simulink model "EScooterBMS"  (R2025b)
settings: Solver=VariableStepAuto  StartTime=0.0  StopTime=3600*20  RelTol=1e-3
InitFcn:
  | EScooterBMS_params
undefined symbols (not defined in the file): balancingThreshold, battery_builder_rtmsupport, CC_Current, currentThreshold, CV_gain, dischargeCurrent, gcbh, initialSOC, initialSOCGuess, noisePower, R, Ts, voltageMin, voltageThreshold
libraries: nesl_utility x6, simulink x5, fl_lib x5, MA1865_1RC_Balancing_lib x2, BatteryBalancing x1, BatteryEstimators x1
settings Model: PacingRate=100  Creator=sturton  LastModifiedBy=sturton

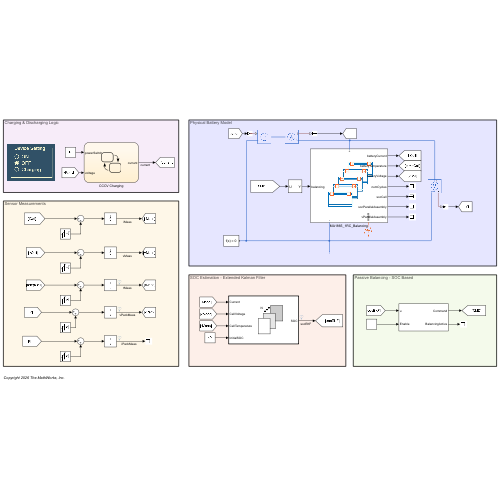
[thumbnail: Simulink's stored preview of the top-level diagram]
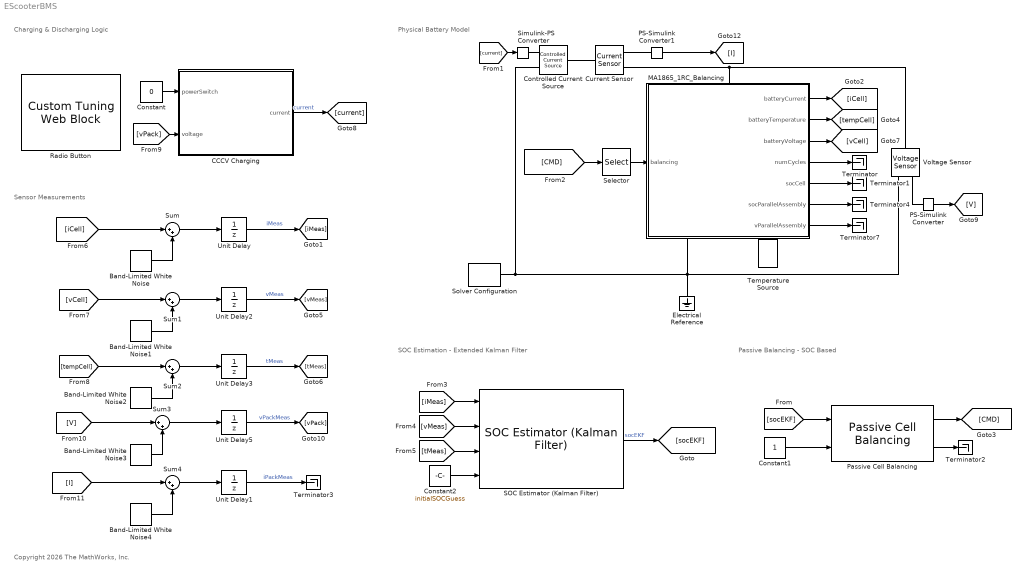
== system EScooterBMS ==
  note: Copyright 2026 The MathWorks, Inc.
  note: Charging & Discharging Logic
  note: Sensor Measurements
  note: SOC Estimation - Extended Kalman Filter
  note: Physical Battery Model
  note: Passive Balancing - SOC Based
  Band-Limited White Noise : simulink/Sources/Band-Limited White Noise  Cov=noisePower  Ts=Ts  seed=[23341]
  Band-Limited White Noise1 : simulink/Sources/Band-Limited White Noise  Cov=noisePower/100;  Ts=Ts  seed=[23341]
  Band-Limited White Noise2 : simulink/Sources/Band-Limited White Noise  Cov=noisePower  Ts=Ts  seed=[23341]
  Band-Limited White Noise3 : simulink/Sources/Band-Limited White Noise  Cov=noisePower/100;  Ts=Ts  seed=[23341]
  Band-Limited White Noise4 : simulink/Sources/Band-Limited White Noise  Cov=noisePower  Ts=Ts  seed=[23341]
  CCCV Charging : Stateflow chart  TreatAsAtomicUnit=on
  Constant : Constant  Value=0
  Constant1 : Constant
  Constant2 : Constant  Value=initialSOCGuess
  Controlled Current Source : fl_lib/Electrical/Electrical Sources/Controlled Current Source
  Current Sensor : fl_lib/Electrical/Electrical Sensors/Current Sensor
  Electrical Reference : fl_lib/Electrical/Electrical Elements/Electrical Reference
  MA1865_1RC_Balancing : Subsystem  LoadFcn=battery_builder_rtmsupport('loadfcn',gcbh);
      settings: CopyFcn=battery_builder_rtmsupport('copyfcn',gcbh);  PreCopyFcn=battery_builder_rtmsupport('precopyfcn',gcbh);  PreDeleteFcn=battery_builder_rtmsupport('predeletefcn',gcbh);  PortSchema="{\"entries\":[{\"content\":{\"sides\":[{\"content\":{\"connectorIds\":[\"LConn1\"]},\"type\":\"ConnectorPlacement.EquallySpacedRectSide\",\"uuid\":\"68ab6467-2481-45d5-b31e-65f7da693cdd\"},{\"content\":{\"connectorIds\":[\"RConn1\",\"RConn2\"],\"side\":\"RIGHT\"},\"type\":\"ConnectorPlacement.EquallySpacedRectSide\",\"uuid\":\"28f8b7ad-849b-43ef-a357-ff2296ceb517\"},{\"content\":{\"connectorIds\":[\"In1\"],\"side\":\"TOP\"},\"type\":\"ConnectorPlacement.EquallySpacedRectSide\",\"uuid\":\"4bc70995-0dac-442d-9c06-590b4a7fbec4\"},{\"content\":{\"connectorIds\":[\"Out1\",\"Out2\",\"Out3\",\"Out4\",\"Out5\",\"Out6\",\"Out7\"],\"side\":\"BOTTOM\"},\"type\":\"ConnectorPlacement.EquallySpacedRectSide\",\"uuid\":\"3fb7c4af-3c1e-4317-a54e-7f7a844b4b32\"}]},\"type\":\"ConnectorPlacement.EquallySpacedConnector\",\"uuid\":\"b72d0926-0e23-41a7-8fa8-9d2afaa8a9c6\"}],\"packageUris\":[\"http://schema.mathworks.com/mf0/Connector/R2020b\"],\"version\":\"1.0\"}"
      mask Display: image('$imagefile')
  PS-Simulink Converter : nesl_utility/PS-Simulink Converter  PhysicalDomain=network_engine_domain  SubClassName=ps_output  LeftPortType=input  RightPortType=output  PseudoPeriodic=off  Frequencies=[]  VectorFormat=inherit  Unit=inherit  AffineConversion=off
  PS-Simulink Converter1 : nesl_utility/PS-Simulink Converter  PhysicalDomain=network_engine_domain  SubClassName=ps_output  LeftPortType=input  RightPortType=output  PseudoPeriodic=off  Frequencies=[]  VectorFormat=inherit  Unit=inherit  AffineConversion=off
  Passive Cell Balancing : BatteryBalancing/Passive Cell Balancing  Threshold=balancingThreshold  HysteresisBand=0  Td_on=1  Td_off=1  Ts=Ts  dataType=double
      settings: LibrarySourceBlock=batt_sl_lib/Cell Balancing/Passive Cell Balancing
  Radio Button : CustomTuningWebBlock  LabelPosition=Hide  ShowInitialText=on  Configuration="{\"components\":[{\"name\":\"RadioButtonStateComponent\",\"settings\":{\"clearedIcon\":{\"size\":[1,1],\"src\":\"data:image\\/svg+xml;base64,PD94bWwgdmVyc2lvbj0iMS4wIiBlbmNvZGluZz0iVVRGLTgiPz4KPHN2ZyBpZD0ic3ZnOCIgeG1sbnM9Imh0dHA6Ly93d3cudzMub3JnLzIwMDAvc3ZnIiB2ZXJzaW9uPSIxLjEiIHhtbG5zOmNjPSJodHRwOi8vY3JlYXRpdmVjb21tb25zLm9yZy9ucyMiIHhtbG5zOmRjPSJodHRwOi8vcHVybC5vcmcvZGMvZWxlbWVudHMvMS4xLyIgeG1sbnM6aW5rc2NhcGU9Imh0dHA6Ly93d3cuaW5rc2NhcGUub3JnL25hbWVzcGFjZXMvaW5rc2NhcGUiIHhtbG5zOnJkZj0iaHR0cDovL3d3dy53My5vcmcvMTk5OS8wMi8yMi1yZGYtc3ludGF4LW5zIyIgeG1sbnM6c29kaXBvZGk9Imh0dHA6Ly9zb2RpcG9kaS5zb3VyY2Vmb3JnZS5uZXQvRFREL3NvZGlwb2RpLTAuZHRkIiB4bWxuczpzdmc9Imh0dHA6Ly93d3cudzMub3JnLzIwMDAvc3ZnIiB2aWV3Qm94PSIwIDAgMzE2LjQgMzE2LjQiPgogIDwhLS0gR2VuZXJhdG9yOiBBZG9iZSBJbGx1c3RyYXRvciAyOS4xLjAsIFNWRyBFeHBvcnQgUGx1Zy1JbiAuIFNWRyBWZXJzaW9uOiAyLjEuMCBCdWlsZCAxNDIpICAtLT4KICA8ZGVmcz4KICAgIDxzdHlsZT4KICAgICAgLnN0MCB7CiAgICAgICAgZmlsbDogbm9uZTsKICAgICAgICBzdHJva2Utd2lkdGg6IDMwcHg7CiAgICAgIH0KCiAgICAgIC5zdDAsIC5zdDEgewogICAgICAgIHN0cm9rZTogI2ZjZmNjNTsKICAgICAgICBzdHJva2UtbWl0ZXJsaW1pdDogMTEuMzsKICAgICAgfQoKICAgICAgLnN0MSB7CiAgICAgICAgZGlzcGxheTogbm9uZTsKICAgICAgICBmaWxsOiAjZmNmY2M1OwogICAgICB9CiAgICA8L3N0eWxlPgogIDwvZGVmcz4KICA8c29kaXBvZGk6bmFtZWR2aWV3IGlkPSJiYXNlIiBib3JkZXJjb2xvcj0iIzY2NjY2NiIgYm9yZGVyb3BhY2l0eT0iMS4wIiBpbmtzY2FwZTpjdXJyZW50LWxheWVyPSJsYXllcjEiIGlua3NjYXBlOmN4PSI0MDAiIGlua3NjYXBlOmN5PSI1NjAiIGlua3NjYXBlOmRvY3VtZW50LXJvdGF0aW9uPSIwIiBpbmtzY2FwZTpkb2N1bWVudC11bml0cz0ibW0iIGlua3NjYXBlOnBhZ2VvcGFjaXR5PSIwLjAiIGlua3NjYXBlOnBhZ2VzaGFkb3c9IjIiIGlua3NjYXBlOndpbmRvdy1oZWlnaHQ9IjEwODEiIGlua3NjYXBlOndpbmRvdy1tYXhpbWl6ZWQ9IjAiIGlua3NjYXBlOndpbmRvdy13aWR0aD0iMTI1MiIgaW5rc2NhcGU6d2luZG93LXg9IjAiIGlua3NjYXBlOndpbmRvdy15PSIyMyIgaW5rc2NhcGU6em9vbT0iMC4zNSIgcGFnZWNvbG9yPSIjZmZmZmZmIiBzaG93Z3JpZD0iZmFsc2UiLz4KICA8Y2lyY2xlIGNsYXNzPSJzdDAiIGN4PSIxNTguMiIgY3k9IjE1OC4yIiByPSIxMzYiLz4KICA8Y2lyY2xlIGNsYXNzPSJzdDEiIGN4PSIxNTguMiIgY3k9IjE1OC4yIiByPSI5OS42Ii8+Cjwvc3ZnPg==\"},\"color\":[0,0,0],\"groupBorderColor\":[252,252,197],\"groupBorderThickness\":\"1\",\"groupTitle\":\"Device Setting\",\"iconOffset\":\"0.5\",\"iconPlacement\":\"left\",\"labelOffset\":[0.2,0.1],\"position\":[0,0,1,1],\"selectedIcon\":{\"size\":[1,1],\"src\":\"data:image\\/svg+xml;base64,PD94bWwgdmVyc2lvbj0iMS4wIiBlbmNvZGluZz0iVVRGLTgiPz4KPHN2ZyBpZD0ic3ZnOCIgeG1sbnM9Imh0dHA6Ly93d3cudzMub3JnLzIwMDAvc3ZnIiB2ZXJzaW9uPSIxLjEiIHhtbG5zOmNjPSJodHRwOi8vY3JlYXRpdmVjb21tb25zLm9yZy9ucyMiIHhtbG5zOmRjPSJodHRwOi8vcHVybC5vcmcvZGMvZWxlbWVudHMvMS4xLyIgeG1sbnM6aW5rc2NhcGU9Imh0dHA6Ly93d3cuaW5rc2NhcGUub3JnL25hbWVzcGFjZXMvaW5rc2NhcGUiIHhtbG5zOnJkZj0iaHR0cDovL3d3dy53My5vcmcvMTk5OS8wMi8yMi1yZGYtc3ludGF4LW5zIyIgeG1sbnM6c29kaXBvZGk9Imh0dHA6Ly9zb2RpcG9kaS5zb3VyY2Vmb3JnZS5uZXQvRFREL3NvZGlwb2RpLTAuZHRkIiB4bWxuczpzdmc9Imh0dHA6Ly93d3cudzMub3JnLzIwMDAvc3ZnIiB2aWV3Qm94PSIwIDAgMzE2LjQgMzE2LjQiPgogIDwhLS0gR2VuZXJhdG9yOiBBZG9iZSBJbGx1c3RyYXRvciAyOS4xLjAsIFNWRyBFeHBvcnQgUGx1Zy1JbiAuIFNWRyBWZXJzaW9uOiAyLjEuMCBCdWlsZCAxNDIpICAtLT4KICA8ZGVmcz4KICAgIDxzdHlsZT4KICAgICAgLnN0MCB7CiAgICAgICAgZmlsbDogI2ZjZmNjNTsKICAgICAgfQoKICAgICAgLnN0MCwgLnN0MSB7CiAgICAgICAgc3Ryb2tlOiAjZmNmY2M1OwogICAgICAgIHN0cm9rZS1taXRlcmxpbWl0OiAxMS4zOwogICAgICB9CgogICAgICAuc3QxIHsKICAgICAgICBmaWxsOiBub25lOwogICAgICAgIHN0cm9rZS13aWR0aDogMzBweDsKICAgICAgfQogICAgPC9zdHlsZT4KICA8L2RlZnM+CiAgPHNvZGlwb2RpOm5hbWVkdmlldyBpZD0iYmFzZSIgYm9yZGVyY29sb3I9IiM2NjY2NjYiIGJvcmRlcm9wYWNpdHk9IjEuMCIgaW5rc2NhcGU6Y3VycmVudC1sYXllcj0ibGF5ZXIxIiBpbmtzY2FwZTpjeD0iNDAwIiBpbmtzY2FwZTpjeT0iNTYwIiBpbmtzY2FwZTpkb2N1bWVudC1yb3RhdGlvbj0iMCIgaW5rc2NhcGU6ZG9jdW1lbnQtdW5pdHM9Im1tIiBpbmtzY2FwZTpwYWdlb3BhY2l0eT0iMC4wIiBpbmtzY2FwZTpwYWdlc2hhZG93PSIyIiBpbmtzY2FwZTp3aW5kb3ctaGVpZ2h0PSIxMDgxIiBpbmtzY2FwZTp3aW5kb3ctbWF4aW1pemVkPSIwIiBpbmtzY2FwZTp3aW5kb3ctd2lkdGg9IjEyNTIiIGlua3NjYXBlOndpbmRvdy14PSIwIiBpbmtzY2FwZTp3aW5kb3cteT0iMjMiIGlua3NjYXBlOnpvb209IjAuMzUiIHBhZ2Vjb2xvcj0iI2ZmZmZmZiIgc2hvd2dyaWQ9ImZhbHNlIi8+CiAgPGNpcmNsZSBjbGFzcz0ic3QxIiBjeD0iMTU4LjIiIGN5PSIxNTguMiIgcj0iMTM2Ii8+CiAgPGNpcmNsZSBjbGFzcz0ic3QwIiBjeD0iMTU4LjIiIGN5PSIxNTguMiIgcj0iOTkuNiIvPgo8L3N2Zz4=\"},\"showGroup\":true,\"states\":[{\"Label\":{\"show\":true,\"text\":{\"content\":\"ON\",\"font\":\"Helvetica\"}},\"Value\":1},{\"Label\":{\"show\":true,\"text\":{\"content\":\"OFF\",\"font\":\"Helvetica\"}},\"Value\":0},{\"Label\":{\"show\":true,\"text\":{\"content\":\"Charging\",\"font\":\"Helvetica\"}},\"Value\":2}]}},{\"name\":\"BackgroundImageComponent\",\"settings\":{\"image\":{\"size\":[146,150],\"src\":\"data:image\\/svg+xml;base64,PD94bWwgdmVyc2lvbj0iMS4wIiBlbmNvZGluZz0iVVRGLTgiPz4KPHN2ZyBpZD0iZnJhbWUiIHhtbG5zPSJodHRwOi8vd3d3LnczLm9yZy8yMDAwL3N2ZyIgdmVyc2lvbj0iMS4xIiB4bWxuczp4bGluaz0iaHR0cDovL3d3dy53My5vcmcvMTk5OS94bGluayIgdmlld0JveD0iMCAwIDM4MC42IDM5MCI+CiAgPCEtLSBHZW5lcmF0b3I6IEFkb2JlIElsbHVzdHJhdG9yIDI5LjEuMCwgU1ZHIEV4cG9ydCBQbHVnLUluIC4gU1ZHIFZlcnNpb246IDIuMS4wIEJ1aWxkIDE0MikgIC0tPgogIDxkZWZzPgogICAgPHN0eWxlPgogICAgICAuc3QwIHsKICAgICAgICBmaWxsOiB1cmwoI3JhZGlhbC1ncmFkaWVudCk7CiAgICAgIH0KCiAgICAgIC5zdDEgewogICAgICAgIGZpbGw6ICM0MjcwODI7CiAgICAgIH0KCiAgICAgIC5zdDIgewogICAgICAgIGZpbGw6ICMwMDJiNDI7CiAgICAgIH0KICAgIDwvc3R5bGU+CiAgICA8cmFkaWFsR3JhZGllbnQgaWQ9InJhZGlhbC1ncmFkaWVudCIgY3g9IjE5MC4zIiBjeT0iLTkzIiBmeD0iMTkwLjMiIGZ5PSItOTMiIHI9IjM3My4xIiBncmFkaWVudFRyYW5zZm9ybT0idHJhbnNsYXRlKDAgMTAyKSBzY2FsZSgxIC0xKSIgZ3JhZGllbnRVbml0cz0idXNlclNwYWNlT25Vc2UiPgogICAgICA8c3RvcCBvZmZzZXQ9IjAiIHN0b3AtY29sb3I9IiMzZTRmNTgiLz4KICAgICAgPHN0b3Agb2Zmc2V0PSIwIiBzdG9wLWNvbG9yPSIjNDQ1NzYxIi8+CiAgICAgIDxzdG9wIG9mZnNldD0iLjIiIHN0b3AtY29sb3I9IiM1NTZhNzYiLz4KICAgICAgPHN0b3Agb2Zmc2V0PSIuMiIgc3RvcC1jb2xvcj0iIzZkODg5NSIvPgogICAgICA8c3RvcCBvZmZzZXQ9Ii40IiBzdG9wLWNvbG9yPSIjOGZiMmMzIi8+CiAgICAgIDxzdG9wIG9mZnNldD0iLjUiIHN0b3AtY29sb3I9IiNiNmU0ZmEiLz4KICAgICAgPHN0b3Agb2Zmc2V0PSIxIiBzdG9wLWNvbG9yPSIjMTU0NjU3Ii8+CiAgICA8L3JhZGlhbEdyYWRpZW50PgogIDwvZGVmcz4KICA8ZyBpZD0iTGF5ZXJfMiI+CiAgICA8ZyBpZD0iTGF5ZXJfMS0yIj4KICAgICAgPHBhdGggaWQ9InBhdGgxMDM4IiBjbGFzcz0ic3QxIiBkPSJNOCw4djM3NS4xaDM2NFY4SDhaTTM2OSw5MCwxMSwxMSIvPgogICAgICA8cGF0aCBpZD0icGF0aDEwNDAiIGNsYXNzPSJzdDAiIGQ9Ik0wLDBsLjYsMzkwaDM4MGwtLjYtMzkwSDBaTTM3MiwzODMuMUg4VjhoMzY0djM3NS4xWiIvPgogICAgPC9nPgogIDwvZz4KICA8cmVjdCBjbGFzcz0ic3QyIiB4PSIxNC44IiB5PSIxNC41IiB3aWR0aD0iMzQ5LjYiIGhlaWdodD0iMzYwLjkiLz4KPC9zdmc+\",\"srcOrientation\":\"Right\"},\"position\":[0,0,1,1],\"scaleMode\":\"0\"}},{\"name\":\"ForegroundImageComponent\",\"settings\":{\"image\":{\"size\":[0,0],\"src\":\"default\",\"srcOrientation\":[]},\"isForeground\":1,\"position\":[0,0,1,1],\"scaleMode\":\"0\"}}],\"derived\":{\"blockParameters\":{\"fixedAspectRatio\":\"on\"}},\"settings\":{\"BindingType\":\"param\",\"backgroundColor\":[0,0,0],\"backgroundOffset\":0,\"enumDataType\":\"\",\"fixedAspectRatio\":\"on\",\"foregroundColor\":[0,0,0],\"showBackgroundColor\":false,\"useEnumDataType\":false,\"version\":\"R2025a\"},\"type\":\"RadioButton\"}"  CustomBackgroundColor="{\"color\":[0,0.16862745098039217,0.25882352941176473],\"show\":true}"
  SOC Estimator (Kalman Filter) : BatteryEstimators/SOC Estimator (Kalman Filter)  CurrentInputPartition=on  filterType=Extended Kalman filter  alpha=1  beta=2  kappa=0  Q=Q  Q_2RC=|  R=R  P0=P0  P0_2RC=[1e-5 0 0; 0 1 0;0 0 1]  Ts=Ts  chargeDynamics=One time-constant dynamics  SOC_vec=SOC_BP  T_vec=Temp_BP  R0_mat=R0  R1_mat=R1  tau1_mat=Tau1  R2_mat=[.0109, .0029, .0013; .0069, .0024, .0012; .0047, .0026, .0013; .0034, .0016, .001; .0033, .0023, .0014; .0033, .0018, .0011; .0028, .0017, .0011]  tau2_mat=[20, 36, 39; 31, 45, 39; 109, 105, 61; 36, 29, 26; 59, 77, 67; 40, 33, 29; 25, 39, 33]  V0_mat=OCV  AH=Capacity  DataType=Inherit: auto
      | [1e-6 0 0;
      | 0 1e-6 0; 0 0 1e-6]
      settings: LibrarySourceBlock=|
      | batt_sl_lib/Estimators/SOC Estimator
      | (Kalman Filter)
  Selector : Selector  InputPortWidth=2  IndexOptions=Index vector (dialog)  Indices=[1 1 1 1 1 2 2 2 2 2]  OutputSizes=1
  Simulink-PS Converter : nesl_utility/Simulink-PS Converter  PhysicalDomain=network_engine_domain  SubClassName=ps_input  LeftPortType=input  RightPortType=output  PseudoPeriodic=off  Frequencies=[]  NoiseDistribution=none  NoiseParameters=[]  Unit=A  AffineConversion=off  FilteringAndDerivatives=provide  SimscapeFilterOrder=1  InputFilterTimeConstant=0.001  UdotUserProvided=0
  Solver Configuration : nesl_utility/Solver Configuration  PhysicalDomain=network_engine_domain  SubClassName=solver  LeftPortType=input  RightPortType=generic  Tones=[]  Harmonics=[]  SimulateNoise=off  Profile=off  UseLocalSampling=off  EnableSwitchedLinearOptims=on  FrequencyDomain=off  UseCCode=off  RelTol=0.001  AbsTol=0.001  MinStep=1e-09  ToWorkspace=off  RevertToSquareIcSolve=off  NumHomotopyIterations=100  PhasorMode=off  PhasorModeNumHarmonics=1  ConsistencySolver=NEWTON_XTOL_AFTER_FTOL  IndexReductionMethod=DerivativeReplacement  DoDC=off  ResidualTolerance=1e-09  ConsistencyTolSource=GLOBAL  ConsistencyAbsTol=0.001  ConsistencyRelTol=0.001  ConsistencyTolFactor=0.001  UseLocalSolver=off  LocalSolverChoice=NE_BACKWARD_EULER_ADVANCER  ResolveIndetEquations=on  FunctionEvalNumThread=1  LocalSolverSampleTime=0.001  DoFixedCost=off  MaxNonlinIter=3  MaxModeIter=2  ComputeImpulses=off  ImpulseIterations=2  LinearAlgebra=auto  LinearAlgebraNumThread=0  EquationFormulation=NE_TIME_EF  DelaysMemoryBudget=1024  AutomaticFiltering=on  FilteringTimeConstant=0.001  PartitionStorageMethod=AS_NEEDED  PartitionMemoryBudget=1024  PartitionMethod=ROBUST  MultibodyUseLocalSolver=off  MultibodyLocalSolverChoice=ODE1  MultibodyLocalSolverSampleTime=0.001
  Sum{,1..4} (5 alike) : Sum  Inputs=|++
  Temperature Source : fl_lib/Thermal/Thermal Sources/Temperature Source  temperature=ambientTemp K
  Terminator{,1..4,7} (6 alike) : Terminator
  Unit Delay : UnitDelay  SampleTime=Ts  HasFrameUpgradeWarning=on
  Unit Delay1 : UnitDelay  SampleTime=Ts  HasFrameUpgradeWarning=on
  Unit Delay2 : UnitDelay  InitialCondition=3.65  SampleTime=Ts  HasFrameUpgradeWarning=on
  Unit Delay3 : UnitDelay  InitialCondition=298.15  SampleTime=Ts  HasFrameUpgradeWarning=on
  Unit Delay5 : UnitDelay  InitialCondition=36.5  SampleTime=Ts  HasFrameUpgradeWarning=on
  Voltage Sensor : fl_lib/Electrical/Electrical Sensors/Voltage Sensor
  wires:
  Band-Limited White Noise1/1 -> Sum1/2
  Band-Limited White Noise/1 -> Sum/2
  [tempCell] -> Sum2/1
  [iMeas] -> SOC Estimator (Kalman Filter)/1
  Unit Delay3/1 -> [tMeas]  "tMeas"
  [tMeas] -> SOC Estimator (Kalman Filter)/3
  [vCell] -> Sum1/1
  [iCell] -> Sum/1
  Constant2/1 -> SOC Estimator (Kalman Filter)/4
  [vMeas] -> SOC Estimator (Kalman Filter)/2
  Band-Limited White Noise2/1 -> Sum2/2
  MA1865_1RC_Balancing/3(batteryVoltage) -> [vCell]
  MA1865_1RC_Balancing/6(socParallelAssembly) -> Terminator4/1
  MA1865_1RC_Balancing/2(batteryTemperature) -> [tempCell]
  MA1865_1RC_Balancing/1(batteryCurrent) -> [iCell]
  MA1865_1RC_Balancing/5(socCell) -> Terminator1/1
  MA1865_1RC_Balancing/4(numCycles) -> Terminator/1
  MA1865_1RC_Balancing/7(vParallelAssembly) -> Terminator7/1
  [CMD] -> Selector/1
  Constant1/1 -> Passive Cell Balancing/2
  Passive Cell Balancing/2 -> Terminator2/1
  SOC Estimator (Kalman Filter)/1 -> [socEKF]  "socEKF"
  [socEKF] -> Passive Cell Balancing/1
  Sum/1 -> Unit Delay/1
  Sum1/1 -> Unit Delay2/1
  Passive Cell Balancing/1 -> [CMD]
  Selector/1 -> MA1865_1RC_Balancing/1(balancing)
  CCCV Charging/1(current) -> [current]  "current"
  [current] -> Simulink-PS Converter/1
  Constant/1 -> CCCV Charging/1(powerSwitch)
  [vPack] -> CCCV Charging/2(voltage)
  Unit Delay/1 -> [iMeas]  "iMeas"
  Unit Delay2/1 -> [vMeas]  "vMeas"
  Sum2/1 -> Unit Delay3/1
  Sum3/1 -> Unit Delay5/1
  Unit Delay5/1 -> [vPack]  "vPackMeas"
  Band-Limited White Noise3/1 -> Sum3/2
  PS-Simulink Converter/1 -> [V]
  [V] -> Sum3/1
  Unit Delay1/1 -> Terminator3/1  "iPackMeas"
  Sum4/1 -> Unit Delay1/1
  Band-Limited White Noise4/1 -> Sum4/2
  PS-Simulink Converter1/1 -> [I]
  [I] -> Sum4/1
  connections:
  Controlled Current Source/RConn2 -- Solver Configuration/RConn1 -- Electrical Reference/LConn1 -- Voltage Sensor/RConn2 -- MA1865_1RC_Balancing/RConn1
  Voltage Sensor/LConn1 -- Current Sensor/RConn2 -- MA1865_1RC_Balancing/LConn1
  Simulink-PS Converter/RConn1 -- Controlled Current Source/RConn1
  MA1865_1RC_Balancing/RConn2 -- Temperature Source/LConn1
  PS-Simulink Converter/LConn1 -- Voltage Sensor/RConn1
  Current Sensor/LConn1 -- Controlled Current Source/LConn1
  PS-Simulink Converter1/LConn1 -- Current Sensor/RConn1

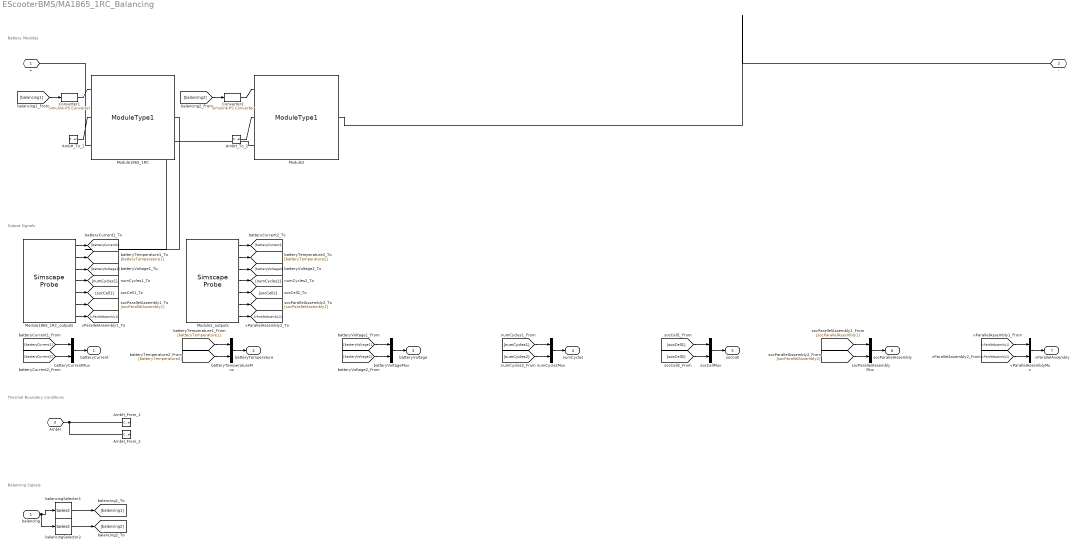
== system EScooterBMS/MA1865_1RC_Balancing ==
  note: Balancing Signals
  note: Thermal Boundary Conditions
  note: Output Signals
  note: Battery Modules
  balancing : Inport  PortDimensions=10
  AmbH_From_1 : ConnectionLabel  Label=ambH_1
  AmbH_From_2 : ConnectionLabel  Label=ambH_2
  AmbH_To_1 : ConnectionLabel  Label=ambH_1
  AmbH_To_2 : ConnectionLabel  Label=ambH_2
  Converter1 : nesl_utility/Simulink-PS Converter  PhysicalDomain=network_engine_domain  SubClassName=ps_input  LeftPortType=input  RightPortType=output  PseudoPeriodic=off  Frequencies=[]  NoiseDistribution=none  NoiseParameters=[]  Unit=1  AffineConversion=off  FilteringAndDerivatives=provide  SimscapeFilterOrder=1  InputFilterTimeConstant=0.001  UdotUserProvided=0
  Converter2 : nesl_utility/Simulink-PS Converter  PhysicalDomain=network_engine_domain  SubClassName=ps_input  LeftPortType=input  RightPortType=output  PseudoPeriodic=off  Frequencies=[]  NoiseDistribution=none  NoiseParameters=[]  Unit=1  AffineConversion=off  FilteringAndDerivatives=provide  SimscapeFilterOrder=1  InputFilterTimeConstant=0.001  UdotUserProvided=0
  Module1865_1RC : MA1865_1RC_Balancing_lib/Modules/ModuleType1  BatteryCapacityCell=ModuleType1.BatteryCapacityCell A*hr  ExtrapolationMethodCell=simscape.enum.extrapolation.nearest  SOCBreakpointsCell=ModuleType1.SOCBreakpointsCell  TemperatureBreakpointsCell=ModuleType1.TemperatureBreakpointsCell K  OpenCircuitVoltageThermalCell=ModuleType1.OpenCircuitVoltageThermalCell V  VoltageRangeCell=ModuleType1.VoltageRangeCell V  ResistanceSOCBreakpointsCell=ModuleType1.ResistanceSOCBreakpointsCell  ResistanceTemperatureBreakpointsCell=ModuleType1.ResistanceTemperatureBreakpointsCell K  R0ThermalCell=ModuleType1.R0ThermalCell Ohm  R1ThermalCell=ModuleType1.R1ThermalCell Ohm  Tau1ThermalCell=ModuleType1.Tau1ThermalCell s  BatteryThermalMassCell=ModuleType1.BatteryThermalMassCell J/K  AmbientResistance=ModuleType1.AmbientResistance K/W  CellBalancingClosedResistance=ModuleType1.CellBalancingClosedResistance Ohm  CellBalancingOpenConductance=ModuleType1.CellBalancingOpenConductance 1/Ohm  CellBalancingThreshold=ModuleType1.CellBalancingThreshold  CellBalancingResistance=ModuleType1.CellBalancingResistance Ohm  P=4  S=5  socCell_specify=on  socCell_priority=High  socCell=initialSOC(1)  socCell_nominal_specify=off  socCell_nominal_value=1  socCell_nominal_unit=1  batteryVoltage_specify=off  batteryVoltage_priority=None  batteryVoltage=0 V  batteryVoltage_nominal_specify=off  batteryVoltage_nominal_value=1  batteryVoltage_nominal_unit=V  batteryCurrent_specify=off  batteryCurrent_priority=None  batteryCurrent=0 A  batteryCurrent_nominal_specify=off  batteryCurrent_nominal_value=1  batteryCurrent_nominal_unit=A  numCycles_specify=off  numCycles_priority=High  numCycles=0  numCycles_nominal_specify=off  numCycles_nominal_value=1  numCycles_nominal_unit=1  batteryTemperature_specify=off  batteryTemperature_priority=High  batteryTemperature=298.15 K  batteryTemperature_nominal_specify=off  batteryTemperature_nominal_value=1  batteryTemperature_nominal_unit=K  vParallelAssembly_specify=off  vParallelAssembly_priority=None  vParallelAssembly=repmat(0, 5, 1) V  vParallelAssembly_nominal_specify=off  vParallelAssembly_nominal_value=1  vParallelAssembly_nominal_unit=V  socParallelAssembly_specify=off  socParallelAssembly_priority=None  socParallelAssembly=repmat(1, 5, 1)  socParallelAssembly_nominal_specify=off  socParallelAssembly_nominal_value=1  socParallelAssembly_nominal_unit=1
      settings: AttributesFormatString=%<socCell_specify>  InternalSimscapePortConfiguration="{\"Bottom\":[{\"id\":\"n\",\"label\":\"-\",\"type\":\"foundation.electrical.electrical\"}],\"Left\":[{\"id\":\"enableCellBalancing\",\"label\":\"CB\",\"type\":\"input\"},{\"id\":\"AmbH\",\"label\":\"AmbH\",\"type\":\"foundation.thermal.thermal\"}],\"Right\":[],\"Top\":[{\"id\":\"p\",\"label\":\"+\",\"type\":\"foundation.electrical.electrical\"}]}"
  Module1865_1RC_outputs : SimscapeProbe  BoundBlock=38  Variables="{\"batteryCurrent\":{\"Probing\":\"ON\"},\"batteryTemperature\":{\"Probing\":\"ON\"},\"batteryVoltage\":{\"Probing\":\"ON\"},\"numCycles\":{\"Probing\":\"ON\"},\"socCell\":{\"Probing\":\"ON\"},\"socParallelAssembly\":{\"Probing\":\"ON\"},\"vParallelAssembly\":{\"Probing\":\"ON\"}}"
  Module2 : MA1865_1RC_Balancing_lib/Modules/ModuleType1  BatteryCapacityCell=ModuleType1.BatteryCapacityCell A*hr  ExtrapolationMethodCell=simscape.enum.extrapolation.nearest  SOCBreakpointsCell=ModuleType1.SOCBreakpointsCell  TemperatureBreakpointsCell=ModuleType1.TemperatureBreakpointsCell K  OpenCircuitVoltageThermalCell=ModuleType1.OpenCircuitVoltageThermalCell V  VoltageRangeCell=ModuleType1.VoltageRangeCell V  ResistanceSOCBreakpointsCell=ModuleType1.ResistanceSOCBreakpointsCell  ResistanceTemperatureBreakpointsCell=ModuleType1.ResistanceTemperatureBreakpointsCell K  R0ThermalCell=ModuleType1.R0ThermalCell Ohm  R1ThermalCell=ModuleType1.R1ThermalCell Ohm  Tau1ThermalCell=ModuleType1.Tau1ThermalCell s  BatteryThermalMassCell=ModuleType1.BatteryThermalMassCell J/K  AmbientResistance=ModuleType1.AmbientResistance K/W  CellBalancingClosedResistance=ModuleType1.CellBalancingClosedResistance Ohm  CellBalancingOpenConductance=ModuleType1.CellBalancingOpenConductance 1/Ohm  CellBalancingThreshold=ModuleType1.CellBalancingThreshold  CellBalancingResistance=ModuleType1.CellBalancingResistance Ohm  P=4  S=5  socCell_specify=on  socCell_priority=High  socCell=initialSOC(2)  socCell_nominal_specify=off  socCell_nominal_value=1  socCell_nominal_unit=1  batteryVoltage_specify=off  batteryVoltage_priority=None  batteryVoltage=0 V  batteryVoltage_nominal_specify=off  batteryVoltage_nominal_value=1  batteryVoltage_nominal_unit=V  batteryCurrent_specify=off  batteryCurrent_priority=None  batteryCurrent=0 A  batteryCurrent_nominal_specify=off  batteryCurrent_nominal_value=1  batteryCurrent_nominal_unit=A  numCycles_specify=off  numCycles_priority=High  numCycles=0  numCycles_nominal_specify=off  numCycles_nominal_value=1  numCycles_nominal_unit=1  batteryTemperature_specify=off  batteryTemperature_priority=High  batteryTemperature=298.15 K  batteryTemperature_nominal_specify=off  batteryTemperature_nominal_value=1  batteryTemperature_nominal_unit=K  vParallelAssembly_specify=off  vParallelAssembly_priority=None  vParallelAssembly=repmat(0, 5, 1) V  vParallelAssembly_nominal_specify=off  vParallelAssembly_nominal_value=1  vParallelAssembly_nominal_unit=V  socParallelAssembly_specify=off  socParallelAssembly_priority=None  socParallelAssembly=repmat(1, 5, 1)  socParallelAssembly_nominal_specify=off  socParallelAssembly_nominal_value=1  socParallelAssembly_nominal_unit=1
      settings: InternalSimscapePortConfiguration="{\"Bottom\":[{\"id\":\"n\",\"label\":\"-\",\"type\":\"foundation.electrical.electrical\"}],\"Left\":[{\"id\":\"enableCellBalancing\",\"label\":\"CB\",\"type\":\"input\"},{\"id\":\"AmbH\",\"label\":\"AmbH\",\"type\":\"foundation.thermal.thermal\"}],\"Right\":[],\"Top\":[{\"id\":\"p\",\"label\":\"+\",\"type\":\"foundation.electrical.electrical\"}]}"
  Module2_outputs : SimscapeProbe  BoundBlock=40  Variables="{\"batteryCurrent\":{\"Probing\":\"ON\"},\"batteryTemperature\":{\"Probing\":\"ON\"},\"batteryVoltage\":{\"Probing\":\"ON\"},\"numCycles\":{\"Probing\":\"ON\"},\"socCell\":{\"Probing\":\"ON\"},\"socParallelAssembly\":{\"Probing\":\"ON\"},\"vParallelAssembly\":{\"Probing\":\"ON\"}}"
  balancingSelector1 : Selector  InputPortWidth=10  IndexOptions=Index vector (dialog)  Indices="[1  2  3  4  5]"  OutputSizes=1
  balancingSelector2 : Selector  InputPortWidth=10  IndexOptions=Index vector (dialog)  Indices="[6   7   8   9  10]"  OutputSizes=1
  batteryCurrentMux : Mux  Inputs=2
  batteryTemperatureMux : Mux  Inputs=2
  batteryVoltageMux : Mux  Inputs=2
  numCyclesMux : Mux  Inputs=2
  socCellMux : Mux  Inputs=2
  socParallelAssemblyMux : Mux  Inputs=2
  vParallelAssemblyMux : Mux  Inputs=2
  + : PMIOPort  Side=Left
  - : PMIOPort  Port=2  Side=Right
  AmbH : PMIOPort  Port=3  Side=Right  ConnectionType=Connection: foundation.thermal.thermal
  batteryCurrent : Outport
  batteryTemperature : Outport  Port=2
  batteryVoltage : Outport  Port=3
  numCycles : Outport  Port=4
  socCell : Outport  Port=5
  socParallelAssembly : Outport  Port=6
  vParallelAssembly : Outport  Port=7
  wires:
  balancingSelector2/1 -> [balancing2]
  [balancing2] -> Converter2/1
  balancingSelector1/1 -> [balancing1]
  balancing/1 -> balancingSelector2/1, balancingSelector1/1
  [balancing1] -> Converter1/1
  [vParallelAssembly2] -> vParallelAssemblyMux/2
  Module2_outputs/7 -> [vParallelAssembly2]
  [socParallelAssembly2] -> socParallelAssemblyMux/2
  Module2_outputs/6 -> [socParallelAssembly2]
  [socCell2] -> socCellMux/2
  Module2_outputs/5 -> [socCell2]
  [numCycles2] -> numCyclesMux/2
  Module2_outputs/4 -> [numCycles2]
  [batteryVoltage2] -> batteryVoltageMux/2
  Module2_outputs/3 -> [batteryVoltage2]
  [batteryTemperature2] -> batteryTemperatureMux/2
  Module2_outputs/2 -> [batteryTemperature2]
  [batteryCurrent2] -> batteryCurrentMux/2
  Module2_outputs/1 -> [batteryCurrent2]
  [vParallelAssembly1] -> vParallelAssemblyMux/1
  vParallelAssemblyMux/1 -> vParallelAssembly/1
  Module1865_1RC_outputs/7 -> [vParallelAssembly1]
  [socParallelAssembly1] -> socParallelAssemblyMux/1
  socParallelAssemblyMux/1 -> socParallelAssembly/1
  Module1865_1RC_outputs/6 -> [socParallelAssembly1]
  [socCell1] -> socCellMux/1
  socCellMux/1 -> socCell/1
  Module1865_1RC_outputs/5 -> [socCell1]
  [numCycles1] -> numCyclesMux/1
  numCyclesMux/1 -> numCycles/1
  Module1865_1RC_outputs/4 -> [numCycles1]
  [batteryVoltage1] -> batteryVoltageMux/1
  batteryVoltageMux/1 -> batteryVoltage/1
  Module1865_1RC_outputs/3 -> [batteryVoltage1]
  [batteryTemperature1] -> batteryTemperatureMux/1
  batteryTemperatureMux/1 -> batteryTemperature/1
  Module1865_1RC_outputs/2 -> [batteryTemperature1]
  [batteryCurrent1] -> batteryCurrentMux/1
  batteryCurrentMux/1 -> batteryCurrent/1
  Module1865_1RC_outputs/1 -> [batteryCurrent1]
  connections:
  AmbH_To_2/LConn1 -- Module2/LConn2
  AmbH_From_2/LConn1 -- AmbH_From_1/LConn1 -- AmbH/RConn1
  AmbH_To_1/LConn1 -- Module1865_1RC/LConn2
  Converter2/RConn1 -- Module2/LConn1
  Converter1/RConn1 -- Module1865_1RC/LConn1
  Module2/RConn1 -- -/RConn1
  Module1865_1RC/LConn3 -- +/RConn1
  Module2/LConn3 -- Module1865_1RC/RConn1

== stateflow chart EScooterBMS/CCCV Charging ==
  state ON
    %
    entry:
    current = dischargeCurrent;
  state Charging
    state CC
      %
      entry:
      current = CC_Current;
    state CV
      %
      during:
      current = current - CV_gain*(voltage - voltageThreshold);
    (default) -> CC
    CC -> CV : [voltage > voltageThreshold]
  state OFF
    %
    entry:
    current = 0;
  ON -> Charging [order 2] : [powerSwitch == 2]
  Charging -> ON [order 2] : [powerSwitch == 1 ]
  ON -> OFF [order 1] : [powerSwitch == 0 || voltage < voltageMin]
  OFF -> ON [order 1] : [powerSwitch == 1 && voltage > 1.1*voltageMin ]
  Charging -> OFF [order 1] : [ powerSwitch == 0 || current < currentThreshold ]
  OFF -> Charging [order 2] : [powerSwitch == 2 && voltage < 0.95*voltageThreshold]
  (default) -> OFF
  data: powerSwitch input; dischargeCurrent parameter; CV_gain parameter; voltageThreshold parameter; CC_Current parameter; currentThreshold parameter; voltageMin parameter; current output; voltage input
